simulink model "MotorDriveThermalTestbench"  (R2024b)
settings: Solver=daessc  StartTime=0.0  StopTime=2400  FixedStep=dt  RelTol=1e-3  AbsTol=1e-3
PreLoadFcn:
  | % Simulation parameters
  | MotorDriveThermalTestBenchParams;
model workspace (MAT data in the model file):
  V_frac_bridge = 0.0437
  V_fract_teeth = 0.9563
values from neighbouring files (symbols this model uses):
  CaseParams = struct()    [InverterThermalParams.m]
  HeatsinkParams = struct()    [InverterThermalParams.m]
undefined symbols (not defined in the file or in its folder): electricDrive, H_AH, H_AL, H_BH, H_BL, H_CH, H_CL, PipeParams, vehicleThermal
libraries: fl_lib x171, ee_lib x31, nesl_utility x28, nesl_utility_internal x12, sdl_lib x6, SimscapeFluids_lib x3, autolibshared x1
(part 2 of 4)

== system MotorDriveThermalTestbench/Motor Cooling/coolantJacket ==
  ControlTsump : fl_lib/Thermal Liquid/Elements/Reservoir (TL)  pressure_spec=foundation.enum.pressure_spec.atmospheric  reservoir_pressure=0.101325 MPa  reservoir_temperature=323.15 K  area=0.01 m^2
  Perfect Insulator : fl_lib/Thermal/Thermal Elements/Perfect Insulator  T_specify=off  T_priority=None  T=293.15 K  T_nominal_specify=off  T_nominal_value=1  T_nominal_unit=K
  Pipe : fl_lib/Thermal Liquid/Elements/Pipe (TL)  length=electricDrive.MotorThermal.ChannelLength mm  area=electricDrive.MotorThermal.ChannelSection mm^2  Dh=electricDrive.MotorThermal.ChannelHydraulicdia mm  length_add=500 mm  roughness=1.5e-5 m  Re_lam=2e+3  Re_tur=4e+3  shape_factor=64  Nu_lam=3.66  dynamic_compressibility=1  inertia=0  p0=1.1 atm  T0=323.15 K  mdot0=0.1 kg/s
  Pump : fl_lib/Thermal Liquid/Sources/Flow Rate Source (TL)  source_type=foundation.enum.constant_controlled.constant  flow_type=foundation.enum.mass_volumetric_flow.mass  mass_flow=pumpFlowRateM kg/s  volumetric_flow=0 m^3/s  power_spec=foundation.enum.power_spec.isentropic  area=pi*20^2 mm^2
      settings: InternalSimscapePortConfiguration="{\"Bottom\":[],\"Left\":[{\"id\":\"A\",\"label\":\"A\",\"type\":\"foundation.thermal_liquid.thermal_liquid\"}],\"Right\":[{\"id\":\"B\",\"label\":\"B\",\"type\":\"foundation.thermal_liquid.thermal_liquid\"}],\"Top\":[]}"
  Thermal Liquid Properties (TL) : SimscapeFluids_lib/Thermal Liquid/Utilities/Thermal Liquid Properties (TL)  fluid_list=fluids.thermal_liquid.utilities.enum.thermal_liquid_fluid_list.ethylene_glycol  concentration_param_EG=fluids.thermal_liquid.utilities.enum.thermal_liquid_concentration.volume_fraction  concentration_param_PG=fluids.thermal_liquid.utilities.enum.thermal_liquid_concentration.volume_fraction  c_mass_SW=3.5e-3  c_mass_EG=0.1  c_mass_PG=0.1  c_mass_GL=0.1  c_vol_EG=0.5  c_vol_PG=0.1  beta_const_EG=2.1791 GPa  beta_const_PG=2.1791 GPa  beta_const_GL=2.1791 GPa  p_min_EG=0.01 MPa  p_min_PG=0.01 MPa  p_min_GL=0.01 MPa  p_max_EG=50 MPa  p_max_PG=50 MPa  p_max_GL=50 MPa  p_atm=0.101325 MPa  properties_range_check=simscape.enum.assert.action.error
  JacketH : PMIOPort  Side=Left
  WindingH : PMIOPort  Port=2  Side=Left
  Ref : PMIOPort  Port=3  Side=Left
  connections:
  ControlTsump/LConn1 -- Thermal Liquid Properties (TL)/RConn1 -- Pump/LConn1
  Pipe/LConn2 -- JacketH/RConn1
  Pipe/RConn1 -- Pump/RConn1
  Pipe/LConn1 -- Ref/RConn1
  WindingH/RConn1 -- Perfect Insulator/LConn1

== system MotorDriveThermalTestbench/Motor Cooling/windingOilJet ==
  note: 1. Learn more about ThermalResistance submodel
  " oilflowRate " : fl_lib/Physical Signals/Sources/PS Constant  constant=electricDrive.MotorThermal.motorOilflow m^3/s
  Heat Exchanger (TL) : SimscapeFluids_lib/Heat Exchangers/Thermal Liquid/Heat Exchanger (TL)  hex_type=fluids.heat_exchangers.enum.FlowArrangement.ParallelCounter  shell_num=1  cross_type=fluids.heat_exchangers.enum.CrossFlowArrangementTL.MixedMixed  NTU_TLU=[.5, 1, 2, 3, 4, 5]  CR_TLU=[0, .25, .5, .75, 1]  eff_TLU=[.3, .3, .3, .3, .3; .6, .55, .5, .47, .43; .85, .76, .68, .61, .55; .94, .83, .72, .65, .58; .98, .86, .75, .66, .58; .99, .86, .75, .66, .58]  R_wall=1.6e-4 K/W  min_flow_area_1=0.01 m^2  Dh_press_1=0.1 m  liquid_volume_1=0.01 m^3  Re_lam_1=2000  Re_tur_1=4000  pressure_loss_spec_1=fluids.heat_exchangers.enum.PressureLossSpec.LossCoeff  pressure_loss_coeff_1=0.1  length_press_1=1 m  length_add_1=0.1 m  roughness_1=15e-6 m  Re_friction_TLU_1=[400, 1000, 1500, 3000, 4000, 6000, 10000, 20000, 40000, 60000, 100000, 100000000]  friction_factor_TLU_1=[.264, .112, .071, .0417, .0387, .0268, .025, .0232, .0226, .022, .0214, .0214]  shape_factor_1=64  Re_Euler_TLU_1=[50, 500, 1000, 2000]  Euler_TLU_1=[4.4505, .6864, .4791, .3755]  heat_transfer_spec_1=fluids.heat_exchangers.enum.HeatCoeffSpec.Constant  heat_transfer_area_1=0.4 m^2  heat_coeff_1=250 W/(K*m^2)  length_heat_1=1 m  Nu_lam_1=3.66  Re_Colburn_TLU_1=[100, 150, 1000]  Colburn_factor_TLU_1=[.019, .013, .002]  Re_Nu_TLU_1=[100, 150, 1000]  Pr_Nu_TLU_1=[1, 10]  Nu_TLU_1=[3.72, 4.21; 3.75, 4.44; 4.21, 7.15]  fouling_factor_1=1e-4 K*m^2/W  min_heat_coeff_1=5 W/(K*m^2)  heat_transfer_area_2=0.4 m^2  fouling_factor_2=1e-4 K*m^2/W  min_heat_coeff_2=5 W/(K*m^2)  dynamic_compressibility_1=simscape.enum.onoff.on  T0_1=298.15 K  p0_1=0.101325 MPa
      settings: InternalSimscapePortConfiguration="{\"Bottom\":[],\"Left\":[{\"id\":\"A1\",\"label\":\"A1\",\"type\":\"foundation.thermal_liquid.thermal_liquid\"},{\"id\":\"B1\",\"label\":\"B1\",\"type\":\"foundation.thermal_liquid.thermal_liquid\"}],\"Right\":[{\"id\":\"H2\",\"label\":\"H2\",\"type\":\"foundation.thermal.thermal\"},{\"id\":\"C2\",\"label\":\"C2\",\"type\":\"input\"},{\"id\":\"HC2\",\"label\":\"HC2\",\"type\":\"input\"}],\"Top\":[]}"
  HeatExHTC : fl_lib/Physical Signals/Sources/PS Constant  constant=300 W/(m^2*K)
  OilHeatCapacity : fl_lib/Physical Signals/Functions/PS Gain  gain=electricDrive.MotorThermal.oilDensity*electricDrive.MotorThermal.oilSpHeat J/(K*m^3)
  Perfect Insulator : fl_lib/Thermal/Thermal Elements/Perfect Insulator  T_specify=off  T_priority=None  T=293.15 K  T_nominal_specify=off  T_nominal_value=1  T_nominal_unit=K
  Pump : fl_lib/Thermal Liquid/Sources/Flow Rate Source (TL)  source_type=foundation.enum.constant_controlled.constant  flow_type=foundation.enum.mass_volumetric_flow.mass  mass_flow=pumpFlowRateM kg/s  volumetric_flow=0 m^3/s  power_spec=foundation.enum.power_spec.isentropic  area=pi*20^2 mm^2
      settings: InternalSimscapePortConfiguration="{\"Bottom\":[],\"Left\":[{\"id\":\"A\",\"label\":\"A\",\"type\":\"foundation.thermal_liquid.thermal_liquid\"}],\"Right\":[{\"id\":\"B\",\"label\":\"B\",\"type\":\"foundation.thermal_liquid.thermal_liquid\"}],\"Top\":[]}"
  Reservoir (TL) : fl_lib/Thermal Liquid/Elements/Reservoir (TL)  pressure_spec=foundation.enum.pressure_spec.atmospheric  reservoir_pressure=0.101325 MPa  reservoir_temperature=TankParams.Temp K  area=0.01 m^2
  Thermal Liquid Properties (TL) : SimscapeFluids_lib/Thermal Liquid/Utilities/Thermal Liquid Properties (TL)  fluid_list=fluids.thermal_liquid.utilities.enum.thermal_liquid_fluid_list.ethylene_glycol  concentration_param_EG=fluids.thermal_liquid.utilities.enum.thermal_liquid_concentration.volume_fraction  concentration_param_PG=fluids.thermal_liquid.utilities.enum.thermal_liquid_concentration.volume_fraction  c_mass_SW=3.5e-3  c_mass_EG=0.1  c_mass_PG=0.1  c_mass_GL=0.1  c_vol_EG=0.5  c_vol_PG=0.1  beta_const_EG=2.1791 GPa  beta_const_PG=2.1791 GPa  beta_const_GL=2.1791 GPa  p_min_EG=0.01 MPa  p_min_PG=0.01 MPa  p_min_GL=0.01 MPa  p_max_EG=50 MPa  p_max_PG=50 MPa  p_max_GL=50 MPa  p_atm=0.101325 MPa  properties_range_check=simscape.enum.assert.action.error
  "ThermalResistance " : Subsystem
      settings: PortSchema="{\"entries\":[{\"content\":{\"sides\":[{\"content\":{\"connectorIds\":[\"LConn1\",\"LConn2\"]},\"type\":\"ConnectorPlacement.EquallySpacedRectSide\",\"uuid\":\"baf5ff6f-2bbb-4e60-9dad-e00baf500c6c\"},{\"content\":{\"connectorIds\":[\"RConn1\"],\"side\":\"RIGHT\"},\"type\":\"ConnectorPlacement.EquallySpacedRectSide\",\"uuid\":\"04d231ab-fa8a-490b-9fb3-01902b632b73\"},{\"content\":{\"connectorIds\":[],\"side\":\"TOP\"},\"type\":\"ConnectorPlacement.EquallySpacedRectSide\",\"uuid\":\"736d11d8-afee-4ef0-b7ea-8bcbaef6669b\"},{\"content\":{\"connectorIds\":[\"RConn2\"],\"side\":\"BOTTOM\"},\"type\":\"ConnectorPlacement.EquallySpacedRectSide\",\"uuid\":\"7a09df8f-6346-484c-a8dd-3bdb74e2d22a\"}]},\"type\":\"ConnectorPlacement.EquallySpacedConnector\",\"uuid\":\"2b9b3d82-05b9-4b26-bdd0-141d56066ae3\"}],\"packageUris\":[\"http://schema.mathworks.com/mf0/Connector/R2020b\"],\"version\":\"1.0\"}"
      mask Display: image('$imagefile'); % Use "Edit Image" on toolstrip to change.
  Variable Thermal Resistance : fl_lib/Thermal/Thermal Elements/Variable Thermal Resistance  R_min=0 K/W  T_specify=off  T_priority=None  T=0 K  T_nominal_specify=off  T_nominal_value=1  T_nominal_unit=K  Q_specify=off  Q_priority=None  Q=0 W  Q_nominal_specify=off  Q_nominal_value=1  Q_nominal_unit=W
      settings: InternalSimscapePortConfiguration="{\"Bottom\":[],\"Left\":[{\"id\":\"A\",\"label\":\"A\",\"type\":\"foundation.thermal.thermal\"},{\"id\":\"R\",\"label\":\"R\",\"type\":\"input\"}],\"Right\":[{\"id\":\"B\",\"label\":\"B\",\"type\":\"foundation.thermal.thermal\"}],\"Top\":[]}"
  avgOilThickness : fl_lib/Physical Signals/Sources/PS Constant  constant=electricDrive.MotorThermal.Oft mm
  windingOD : fl_lib/Physical Signals/Sources/PS Constant  constant=electricDrive.MotorThermal.ODpcd*1e-3 m
  JacketH : PMIOPort  Side=Left
  WindingH : PMIOPort  Port=2  Side=Left
  Ref : PMIOPort  Port=3  Side=Left
  connections:
  Variable Thermal Resistance/RConn1 -- Heat Exchanger (TL)/RConn1
  Variable Thermal Resistance/LConn1 -- WindingH/RConn1
  " oilflowRate "/RConn1 -- OilHeatCapacity/LConn1 -- "ThermalResistance "/RConn2
  avgOilThickness/RConn1 -- "ThermalResistance "/LConn1
  windingOD/RConn1 -- "ThermalResistance "/LConn2
  Variable Thermal Resistance/LConn2 -- "ThermalResistance "/RConn1
  Ref/RConn1 -- Heat Exchanger (TL)/LConn2
  Reservoir (TL)/LConn1 -- Thermal Liquid Properties (TL)/RConn1 -- Pump/LConn1
  Pump/RConn1 -- Heat Exchanger (TL)/LConn1
  HeatExHTC/RConn1 -- Heat Exchanger (TL)/RConn3
  OilHeatCapacity/RConn1 -- Heat Exchanger (TL)/RConn2
  JacketH/RConn1 -- Perfect Insulator/LConn1

== system MotorDriveThermalTestbench/TemperatureLimits/Thermal fault Logic Inverter ==
  tc : Inport
  tm : Inport  Port=2
  CoilTempLimit : Constant  Value=IGBTlim
  Gain : Gain  OutDataTypeStr=double
  MagnetTempL imit : Constant  Value=DiodeLim
  MinMax : MinMax  Function=max  Inputs=2
  Relational Operator : RelationalOperator  OutDataTypeStr=boolean  RndMeth=Simplest  InputSameDT=off
  Relational Operator1 : RelationalOperator  OutDataTypeStr=boolean  RndMeth=Simplest  InputSameDT=off
  Unit Delay : UnitDelay  SampleTime=-1  HasFrameUpgradeWarning=on
  Unit Delay1 : UnitDelay  SampleTime=-1  HasFrameUpgradeWarning=on
  F : Outport
  wires:
  Relational Operator/1 -> MinMax/1
  MagnetTempL imit/1 -> Relational Operator1/2
  Relational Operator1/1 -> MinMax/2
  CoilTempLimit/1 -> Relational Operator/2
  Gain/1 -> F/1
  MinMax/1 -> Gain/1
  Unit Delay/1 -> Relational Operator/1
  tc/1 -> Unit Delay/1
  tm/1 -> Unit Delay1/1
  Unit Delay1/1 -> Relational Operator1/1

== system MotorDriveThermalTestbench/TemperatureLimits/Thermal fault Logic Motor ==
  tc : Inport
  tm : Inport  Port=2
  CoilTempLimit : Constant  Value=coilTLim
  Gain : Gain  OutDataTypeStr=double
  MagnetTempL imit : Constant  Value=MagTLim
  MinMax : MinMax  Function=max  Inputs=2
  Relational Operator : RelationalOperator  OutDataTypeStr=boolean  RndMeth=Simplest  InputSameDT=off
  Relational Operator1 : RelationalOperator  OutDataTypeStr=boolean  RndMeth=Simplest  InputSameDT=off
  Unit Delay : UnitDelay  SampleTime=-1  HasFrameUpgradeWarning=on
  Unit Delay1 : UnitDelay  SampleTime=-1  HasFrameUpgradeWarning=on
  F : Outport
  wires:
  Relational Operator/1 -> MinMax/1
  MagnetTempL imit/1 -> Relational Operator1/2
  Relational Operator1/1 -> MinMax/2
  CoilTempLimit/1 -> Relational Operator/2
  Gain/1 -> F/1
  MinMax/1 -> Gain/1
  Unit Delay/1 -> Relational Operator/1
  tc/1 -> Unit Delay/1
  tm/1 -> Unit Delay1/1
  Unit Delay1/1 -> Relational Operator1/1

== system MotorDriveThermalTestbench/Test Env N Controls/Motor speed N test environment ==
  VehSpd : Inport
  Motor Speed Reference : Subsystem
  Test Environment : Subsystem
  BrakeSig : Outport
  MtrSpdRef : Outport  Port=2
  wires:
  Test Environment/1(BrakeSig) -> BrakeSig/1
  VehSpd/1 -> Test Environment/1(tgtVspd), Motor Speed Reference/1(VSpd)
  Motor Speed Reference/1(MtrSpdRef) -> MtrSpdRef/1

== system MotorDriveThermalTestbench/Test Env N Controls/Speed Controller ==
  Spd : Inport  Unit=rpm
      settings: AttributesFormatString=%<Unit>
  SpdRef : Inport  Port=2  Unit=rpm
      settings: AttributesFormatString=%<Unit>
  Ki : Gain  Gain=electricDrive.PmsmControlParams.Kp_omega
  Kp : Gain  Gain=electricDrive.PmsmControlParams.Ki_omega
  Limits [-40,40] : Integrator  LimitOutput=on  UpperSaturationLimit=40  LowerSaturationLimit=-40
  Saturation : Saturate  UpperLimit=electricDrive.Tmax  LowerLimit=-electricDrive.Tmax
      settings: AttributesFormatString=|
      | %<UpperLimit>
      | %<LowerLimit>
  Sum : Sum  Inputs=-+|
  Sum1 : Sum  Inputs=++|
  Transfer Fcn : TransferFcn  Denominator=[0.1 1]
  TrqCmd : Outport  Unit=N*m  VectorParamsAs1DForOutWhenUnconnected=off
      settings: AttributesFormatString=%<Unit>
  wires:
  Saturation/1 -> TrqCmd/1
  Limits [-40,40]/1 -> Sum1/1
  Kp/1 -> Sum1/2
  Ki/1 -> Limits [-40,40]/1
  Sum/1 -> Kp/1, Ki/1
  Sum1/1 -> Saturation/1
  SpdRef/1 -> Sum/2
  Spd/1 -> Transfer Fcn/1
  Transfer Fcn/1 -> Sum/1

== system MotorDriveThermalTestbench/EM/Air_HTC_calculation/Rotor side  HTC ==
  PS Add : fl_lib/Physical Signals/Functions/PS Add
  PS Constant : fl_lib/Physical Signals/Sources/PS Constant  constant=8.1387 rad/s
  PS Gain1 : fl_lib/Physical Signals/Functions/PS Gain  gain=2.217 W*s/(m^2*K*rad)
  PS Gain2 : fl_lib/Physical Signals/Functions/PS Gain  gain=0.0265
  w : PMIOPort  Side=Left
  HTC : PMIOPort  Port=2  Side=Right
  connections:
  PS Constant/RConn1 -- PS Add/LConn2
  PS Gain2/RConn1 -- PS Add/LConn1
  PS Gain1/LConn1 -- PS Add/RConn1
  PS Gain1/RConn1 -- HTC/RConn1
  PS Gain2/LConn1 -- w/RConn1

== system MotorDriveThermalTestbench/EM/Air_HTC_calculation/Rotor_Taylor_Couette  HTC ==
  PS Add : fl_lib/Physical Signals/Functions/PS Add
  PS Constant : fl_lib/Physical Signals/Sources/PS Constant  constant=8.1387 rad/s
  PS Gain : fl_lib/Physical Signals/Functions/PS Gain  gain=2.667e-6 s/rad
  PS Gain1 : fl_lib/Physical Signals/Functions/PS Gain  gain=1 W/(m^2*K)
  PS Gain2 : fl_lib/Physical Signals/Functions/PS Gain  gain=0.0265
  PS-Simulink Converter : nesl_utility/PS-Simulink Converter  PhysicalDomain=network_engine_domain  SubClassName=ps_output  LeftPortType=input  RightPortType=output  PseudoPeriodic=off  Frequencies=[]  VectorFormat=inherit  Unit=inherit  AffineConversion=off
  Scope : Scope
  w : PMIOPort  Side=Left
  HTC_TC : PMIOPort  Port=2  Side=Right
  wires:
  PS-Simulink Converter/1 -> Scope/1
  connections:
  PS Add/RConn1 -- PS Gain/LConn1
  PS Constant/RConn1 -- PS Add/LConn2
  PS Gain2/RConn1 -- PS Add/LConn1
  HTC_TC/RConn1 -- PS-Simulink Converter/LConn1 -- PS Gain1/RConn1
  w/RConn1 -- PS Gain2/LConn1
  PS Gain/RConn1 -- PS Gain1/LConn1

== system MotorDriveThermalTestbench/EM/Loss Estimation/Copper Loss  ==
  PS Constant : fl_lib/Physical Signals/Sources/PS Constant  constant=0.0103 Ohm
  PS Gain : fl_lib/Physical Signals/Functions/PS Gain  gain=1
  PS Math Function : fl_lib/Physical Signals/Functions/PS Math Function  fcn_choice=foundation.enum.math_function.square  v=1
  PS Product : fl_lib/Physical Signals/Functions/PS Product
  Current : PMIOPort  Side=Left
  I2R : PMIOPort  Port=2  Side=Right
  connections:
  I2R/RConn1 -- PS Gain/RConn1
  PS Product/RConn1 -- PS Gain/LConn1
  PS Math Function/RConn1 -- PS Product/LConn1
  PS Constant/RConn1 -- PS Product/LConn2
  PS Math Function/LConn1 -- Current/RConn1

== system MotorDriveThermalTestbench/EM/Loss Estimation/Iron Loss ==
  PS Gain : fl_lib/Physical Signals/Functions/PS Gain  gain=electricDrive.MotorThermal.vFractBridge*0.4
  PS Gain1 : fl_lib/Physical Signals/Functions/PS Gain  gain=electricDrive.MotorThermal.vFractTooth*1.1
  PS Subtract : fl_lib/Physical Signals/Functions/PS Subtract
  MotH : PMIOPort  Side=Left
  I2R : PMIOPort  Port=2  Side=Left
  rt : PMIOPort  Port=3  Side=Right
  st : PMIOPort  Port=4  Side=Right
  connections:
  PS Gain1/RConn1 -- st/RConn1
  PS Gain/RConn1 -- rt/RConn1
  PS Gain1/LConn1 -- PS Gain/LConn1 -- PS Subtract/RConn1
  I2R/RConn1 -- PS Subtract/LConn2
  MotH/RConn1 -- PS Subtract/LConn1

== system MotorDriveThermalTestbench/EM/Loss Estimation/Subsystem ==
  Heat Flow Rate Sensor : fl_lib/Thermal/Thermal Sensors/Heat Flow Rate Sensor
  Temperature Source : fl_lib/Thermal/Thermal Sources/Temperature Source  temperature=298.15 K
  Hmot : PMIOPort  Side=Left
  MotH : PMIOPort  Port=2  Side=Right
  connections:
  Temperature Source/LConn1 -- Heat Flow Rate Sensor/RConn2
  Hmot/RConn1 -- Heat Flow Rate Sensor/LConn1
  MotH/RConn1 -- Heat Flow Rate Sensor/RConn1

== system MotorDriveThermalTestbench/EM/Subsystem1/Sensing wMotor ==
  PS-Simulink Converter : nesl_utility/PS-Simulink Converter  PhysicalDomain=network_engine_domain  SubClassName=ps_output  LeftPortType=input  RightPortType=output  PseudoPeriodic=off  Frequencies=[]  VectorFormat=1-D array  Unit=rpm  AffineConversion=off
  PS : PMIOPort  Side=Left
  SL : Outport  VectorParamsAs1DForOutWhenUnconnected=off
  wires:
  PS-Simulink Converter/1 -> SL/1
  connections:
  PS/RConn1 -- PS-Simulink Converter/LConn1

== system MotorDriveThermalTestbench/EM/Temperature/Bus ==
  Bus Creator : BusCreator  Inputs=2
  PS-Simulink Converter : nesl_utility/PS-Simulink Converter  PhysicalDomain=network_engine_domain  SubClassName=ps_output  LeftPortType=input  RightPortType=output  PseudoPeriodic=off  Frequencies=[]  VectorFormat=inherit  Unit=inherit  AffineConversion=off
  PS-Simulink Converter1 : nesl_utility/PS-Simulink Converter  PhysicalDomain=network_engine_domain  SubClassName=ps_output  LeftPortType=input  RightPortType=output  PseudoPeriodic=off  Frequencies=[]  VectorFormat=inherit  Unit=inherit  AffineConversion=off
  " " : PMIOPort  Side=Left
  "  " : PMIOPort  Port=2  Side=Left
  "   " : Outport
  wires:
  Bus Creator/1 -> "   "/1
  PS-Simulink Converter/1 -> Bus Creator/1  "Tmag"
  PS-Simulink Converter1/1 -> Bus Creator/2  "Tcoil"
  connections:
  " "/RConn1 -- PS-Simulink Converter/LConn1
  "  "/RConn1 -- PS-Simulink Converter1/LConn1

== system MotorDriveThermalTestbench/EM/Temperature/Rotor Thermal Block ==
  Conductive Heat Transfer : fl_lib/Thermal/Thermal Elements/Conductive Heat Transfer  thermal_type=foundation.enum.ConstantVariableTabulated.Constant  wall_geometry=foundation.enum.ConductionWallGeometry.Cylindrical  area=1e-4 m^2  thickness=0.1 m  d_in=0.005 m  d_out=rotor_od m  L=rotorStackLength m  th_cond_min=10 W/(K*m)  th_cond=IronThConductivity W/(K*m)  th_cond_TLU=[413, 401, 392, 383, 371, 357, 342] W/(K*m)  temp_TLU=[200, 273, 400, 600, 800, 1000, 1200] K  T_specify=off  T_priority=None  T=0 K  T_nominal_specify=off  T_nominal_value=1  T_nominal_unit=K  Q_specify=off  Q_priority=None  Q=0 W  Q_nominal_specify=off  Q_nominal_value=1  Q_nominal_unit=W
  Convective Heat Transfer : fl_lib/Thermal/Thermal Elements/Convective Heat Transfer  thermal_type=foundation.enum.constant_variable.variable  area=RotorAreaCyl m^2  heat_tr_coeff=10 W/(K*m^2)  min_heat_tr_coeff=1e-3 W/(K*m^2)  T_specify=off  T_priority=None  T=0 K  T_nominal_specify=off  T_nominal_value=1  T_nominal_unit=K  Q_specify=off  Q_priority=None  Q=0 W  Q_nominal_specify=off  Q_nominal_value=1  Q_nominal_unit=W
      settings: InternalSimscapePortConfiguration="{\"Bottom\":[],\"Left\":[{\"id\":\"A\",\"label\":\"A\",\"type\":\"foundation.thermal.thermal\"},{\"id\":\"var_heat_tr_coeff\",\"label\":\"K\",\"type\":\"input\"}],\"Right\":[{\"id\":\"B\",\"label\":\"B\",\"type\":\"foundation.thermal.thermal\"}],\"Top\":[]}"
  Convective Heat Transfer1 : fl_lib/Thermal/Thermal Elements/Convective Heat Transfer  thermal_type=foundation.enum.constant_variable.variable  area=RotorAreaER m^2  heat_tr_coeff=20 W/(K*m^2)  min_heat_tr_coeff=1e-3 W/(K*m^2)  T_specify=off  T_priority=None  T=0 K  T_nominal_specify=off  T_nominal_value=1  T_nominal_unit=K  Q_specify=off  Q_priority=None  Q=0 W  Q_nominal_specify=off  Q_nominal_value=1  Q_nominal_unit=W
      settings: InternalSimscapePortConfiguration="{\"Bottom\":[],\"Left\":[{\"id\":\"A\",\"label\":\"A\",\"type\":\"foundation.thermal.thermal\"},{\"id\":\"var_heat_tr_coeff\",\"label\":\"K\",\"type\":\"input\"}],\"Right\":[{\"id\":\"B\",\"label\":\"B\",\"type\":\"foundation.thermal.thermal\"}],\"Top\":[]}"
  Heat Flow Source : fl_lib/Thermal/Thermal Sources/Controlled Heat Flow Rate Source
  "Magnet_Temperature " : fl_lib/Thermal/Thermal Elements/Thermal Mass  mass_type=foundation.enum.constant_variable.constant  mass=Bridgemass kg  sp_heat=IronSpHeat J/(K*kg)  mass_min=1e-6 kg  num_ports=foundation.enum.numPorts2.one  m_specify=off  m_priority=High  m=1 kg  m_nominal_specify=off  m_nominal_value=1  m_nominal_unit=kg  T_specify=on  T_priority=High  T=InitTemp K  T_nominal_specify=off  T_nominal_value=1  T_nominal_unit=K  Q_specify=off  Q_priority=None  Q=0 W  Q_nominal_specify=off  Q_nominal_value=1  Q_nominal_unit=W
  MotorHousingTemperature : fl_lib/Thermal/Thermal Sources/Temperature Source  temperature=90 degC
  Rotor Back Iron : fl_lib/Thermal/Thermal Elements/Thermal Mass  mass_type=foundation.enum.constant_variable.constant  mass=RotorBackIronMass kg  sp_heat=IronSpHeat J/(K*kg)  mass_min=1e-6 kg  num_ports=foundation.enum.numPorts2.one  m_specify=off  m_priority=High  m=1 kg  m_nominal_specify=off  m_nominal_value=1  m_nominal_unit=kg  T_specify=on  T_priority=High  T=InitTemp K  T_nominal_specify=off  T_nominal_value=1  T_nominal_unit=K  Q_specify=off  Q_priority=None  Q=0 W  Q_nominal_specify=off  Q_nominal_value=1  Q_nominal_unit=W
  Sensor : Subsystem
  Thermal Reference : fl_lib/Thermal/Thermal Elements/Thermal Reference
  H_rot : PMIOPort  Side=Right
  HTC_AG : PMIOPort  Port=2  Side=Right
  HTC_ER : PMIOPort  Port=3  Side=Right
  Magnet Temp : PMIOPort  Port=4  Side=Left
  connections:
  Magnet Temp/RConn1 -- Sensor/RConn1
  H_rot/RConn1 -- Heat Flow Source/RConn1
  HTC_ER/RConn1 -- Convective Heat Transfer1/LConn2
  HTC_AG/RConn1 -- Convective Heat Transfer/LConn2
  Convective Heat Transfer/LConn1 -- Sensor/LConn1 -- Conductive Heat Transfer/LConn1 -- "Magnet_Temperature "/LConn1 -- Heat Flow Source/LConn1
  MotorHousingTemperature/LConn1 -- Convective Heat Transfer1/RConn1 -- Convective Heat Transfer/RConn1
  Rotor Back Iron/LConn1 -- Convective Heat Transfer1/LConn1 -- Conductive Heat Transfer/RConn1
  Thermal Reference/LConn1 -- Heat Flow Source/RConn2

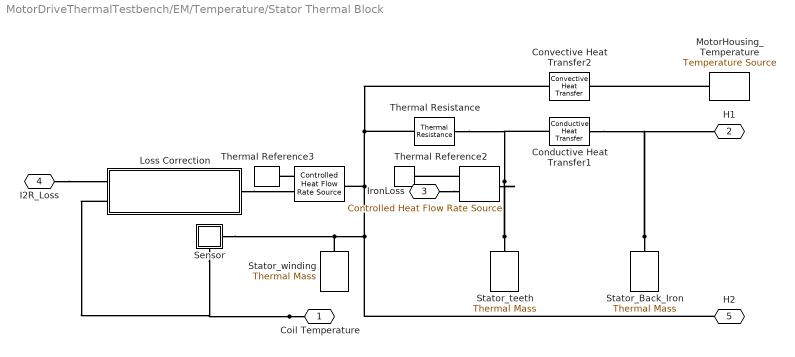
== system MotorDriveThermalTestbench/EM/Temperature/Stator Thermal Block ==
  " " : fl_lib/Thermal/Thermal Sources/Controlled Heat Flow Rate Source
  "  " : fl_lib/Thermal/Thermal Sources/Controlled Heat Flow Rate Source
  Conductive Heat Transfer1 : fl_lib/Thermal/Thermal Elements/Conductive Heat Transfer  thermal_type=foundation.enum.ConstantVariableTabulated.Constant  wall_geometry=foundation.enum.ConductionWallGeometry.Cylindrical  area=1e-4 m^2  thickness=0.1 m  d_in=StatorRootDia m  d_out=stator_od m  L=rotorStackLength m  th_cond_min=10 W/(K*m)  th_cond=50 W/(K*m)  th_cond_TLU=[413, 401, 392, 383, 371, 357, 342] W/(K*m)  temp_TLU=[200, 273, 400, 600, 800, 1000, 1200] K  T_specify=off  T_priority=None  T=0 K  T_nominal_specify=off  T_nominal_value=1  T_nominal_unit=K  Q_specify=off  Q_priority=None  Q=0 W  Q_nominal_specify=off  Q_nominal_value=1  Q_nominal_unit=W
  Convective Heat Transfer2 : fl_lib/Thermal/Thermal Elements/Convective Heat Transfer  thermal_type=foundation.enum.constant_variable.constant  area=StatorWindingOhArea m^2  heat_tr_coeff=1 W/(K*m^2)  min_heat_tr_coeff=1e-3 W/(K*m^2)  T_specify=off  T_priority=None  T=0 K  T_nominal_specify=off  T_nominal_value=1  T_nominal_unit=K  Q_specify=off  Q_priority=None  Q=0 W  Q_nominal_specify=off  Q_nominal_value=1  Q_nominal_unit=W
  Loss Correction : Subsystem
  MotorHousing_Temperature : fl_lib/Thermal/Thermal Sources/Temperature Source  temperature=90 degC
  Sensor : Subsystem
      settings: PortSchema="{\"entries\":[{\"content\":{\"sides\":[{\"content\":{\"connectorIds\":[\"LConn1\"]},\"type\":\"ConnectorPlacement.EquallySpacedRectSide\",\"uuid\":\"2a9c4c46-5e98-4ad3-ac1b-1643fab919e9\"},{\"content\":{\"connectorIds\":[],\"side\":\"RIGHT\"},\"type\":\"ConnectorPlacement.EquallySpacedRectSide\",\"uuid\":\"818e06c0-624d-478e-bbcc-fcb04ee6018d\"},{\"content\":{\"connectorIds\":[],\"side\":\"TOP\"},\"type\":\"ConnectorPlacement.EquallySpacedRectSide\",\"uuid\":\"5528f141-53ee-42de-bb84-2bf943b57dce\"},{\"content\":{\"connectorIds\":[\"RConn1\"],\"side\":\"BOTTOM\"},\"type\":\"ConnectorPlacement.EquallySpacedRectSide\",\"uuid\":\"84eb734e-86a3-4614-b5bf-5af47052b8ad\"}]},\"type\":\"ConnectorPlacement.EquallySpacedConnector\",\"uuid\":\"b22b55cd-2470-4ac9-8f94-59072ebe807a\"}],\"packageUris\":[\"http://schema.mathworks.com/mf0/Connector/R2020b\"],\"version\":\"1.0\"}"
  Stator_Back_Iron : fl_lib/Thermal/Thermal Elements/Thermal Mass  mass_type=foundation.enum.constant_variable.constant  mass=StatorBackIronMass kg  sp_heat=IronSpHeat J/(K*kg)  mass_min=1e-6 kg  num_ports=foundation.enum.numPorts2.one  m_specify=off  m_priority=High  m=1 kg  m_nominal_specify=off  m_nominal_value=1  m_nominal_unit=kg  T_specify=on  T_priority=High  T=InitTemp K  T_nominal_specify=off  T_nominal_value=1  T_nominal_unit=K  Q_specify=off  Q_priority=None  Q=0 W  Q_nominal_specify=off  Q_nominal_value=1  Q_nominal_unit=W
  Stator_teeth : fl_lib/Thermal/Thermal Elements/Thermal Mass  mass_type=foundation.enum.constant_variable.constant  mass=GrossToothMass kg  sp_heat=IronSpHeat J/(K*kg)  mass_min=1e-6 kg  num_ports=foundation.enum.numPorts2.one  m_specify=off  m_priority=High  m=1 kg  m_nominal_specify=off  m_nominal_value=1  m_nominal_unit=kg  T_specify=on  T_priority=High  T=InitTemp K  T_nominal_specify=off  T_nominal_value=1  T_nominal_unit=K  Q_specify=off  Q_priority=None  Q=0 W  Q_nominal_specify=off  Q_nominal_value=1  Q_nominal_unit=W
  Stator_winding : fl_lib/Thermal/Thermal Elements/Thermal Mass  mass_type=foundation.enum.constant_variable.constant  mass=WindingMass kg  sp_heat=CopperSpHeat J/(K*kg)  mass_min=1e-6 kg  num_ports=foundation.enum.numPorts2.one  m_specify=off  m_priority=High  m=1 kg  m_nominal_specify=off  m_nominal_value=1  m_nominal_unit=kg  T_specify=on  T_priority=High  T=InitTemp K  T_nominal_specify=off  T_nominal_value=1  T_nominal_unit=K  Q_specify=off  Q_priority=None  Q=0 W  Q_nominal_specify=off  Q_nominal_value=1  Q_nominal_unit=W
  Thermal Reference2 : fl_lib/Thermal/Thermal Elements/Thermal Reference
  Thermal Reference3 : fl_lib/Thermal/Thermal Elements/Thermal Reference
  Thermal Resistance : fl_lib/Thermal/Thermal Elements/Thermal Resistance  resistance=0.1 K/W  T_specify=off  T_priority=None  T=0 K  T_nominal_specify=off  T_nominal_value=1  T_nominal_unit=K  Q_specify=off  Q_priority=None  Q=0 W  Q_nominal_specify=off  Q_nominal_value=1  Q_nominal_unit=W
  Coil Temperature : PMIOPort  Side=Left
  H1 : PMIOPort  Port=2  Side=Left
  IronLoss : PMIOPort  Port=3  Side=Right
  I2R_Loss : PMIOPort  Port=4  Side=Right
  H2 : PMIOPort  Port=5  Side=Left
  connections:
  I2R_Loss/RConn1 -- Loss Correction/LConn1
  Coil Temperature/RConn1 -- Loss Correction/LConn2 -- Sensor/LConn1
  Loss Correction/RConn1 -- "  "/RConn1
  IronLoss/RConn1 -- " "/RConn1
  " "/RConn2 -- Thermal Reference2/LConn1
  "  "/RConn2 -- Thermal Reference3/LConn1
  MotorHousing_Temperature/LConn1 -- Convective Heat Transfer2/RConn1
  Sensor/RConn1 -- "  "/LConn1 -- Thermal Resistance/RConn1 -- Convective Heat Transfer2/LConn1 -- H2/RConn1 -- Stator_winding/LConn1
  Stator_teeth/LConn1 -- Thermal Resistance/LConn1 -- Conductive Heat Transfer1/LConn1 -- " "/LConn1
  Stator_Back_Iron/LConn1 -- H1/RConn1 -- Conductive Heat Transfer1/RConn1

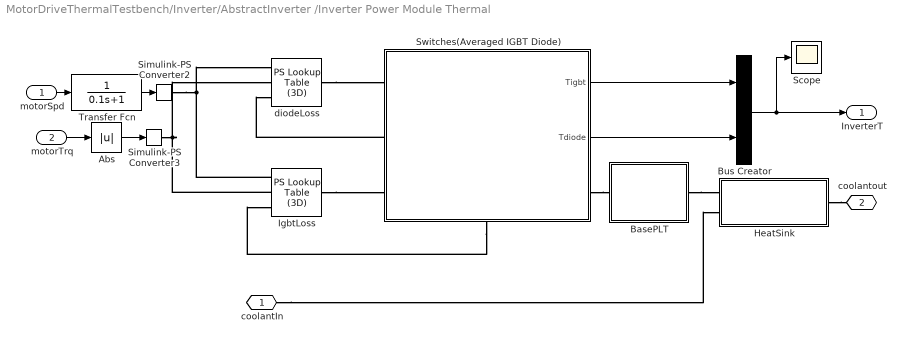
== system MotorDriveThermalTestbench/Inverter/AbstractInverter /Inverter Power Module Thermal ==
  motorSpd : Inport
  motorTrq : Inport  Port=2
  Abs : Abs  SaturateOnIntegerOverflow=off
  BasePLT : Subsystem
  Bus Creator : BusCreator  Inputs=2
  HeatSink : Subsystem
  IgbtLoss : fl_lib/Physical Signals/Lookup Tables/PS Lookup Table (3D)  x1=electricDrive.motor_loss_map.spMat rpm  x2=electricDrive.motor_loss_map.tqMat N*m  x3=[25,125, 175]+273.15 K  f=electricDrive.inverter_loss_map.lossMatIgbt  interp_method=simscape.enum.interpolation.linear  extrap_method=simscape.enum.extrapolation.linear
      settings: InternalSimscapePortConfiguration="{\"Bottom\":[],\"Left\":[{\"id\":\"I1\",\"label\":\"x1\",\"type\":\"input\"},{\"id\":\"I2\",\"label\":\"x2\",\"type\":\"input\"},{\"id\":\"I3\",\"label\":\"x3\",\"type\":\"input\"}],\"Right\":[{\"id\":\"O\",\"label\":\"f\",\"type\":\"output\"}],\"Top\":[]}"
  Scope : Scope
  Simulink-PS Converter2 : nesl_utility/Simulink-PS Converter  PhysicalDomain=network_engine_domain  SubClassName=ps_input  LeftPortType=input  RightPortType=output  PseudoPeriodic=off  Frequencies=[]  NoiseDistribution=none  NoiseParameters=[]  Unit=rpm  AffineConversion=off  FilteringAndDerivatives=provide  SimscapeFilterOrder=1  InputFilterTimeConstant=0.001  UdotUserProvided=0
  Simulink-PS Converter3 : nesl_utility/Simulink-PS Converter  PhysicalDomain=network_engine_domain  SubClassName=ps_input  LeftPortType=input  RightPortType=output  PseudoPeriodic=off  Frequencies=[]  NoiseDistribution=none  NoiseParameters=[]  Unit=N*m  AffineConversion=off  FilteringAndDerivatives=provide  SimscapeFilterOrder=1  InputFilterTimeConstant=0.001  UdotUserProvided=0
  Switches(Averaged IGBT Diode) : Subsystem
      settings: PortSchema="{\"entries\":[{\"content\":{\"sides\":[{\"content\":{\"connectorIds\":[\"Out1\",\"Out2\",\"LConn1\"]},\"type\":\"ConnectorPlacement.EquallySpacedRectSide\",\"uuid\":\"c466717f-a559-4c42-b6dd-2de508982627\"},{\"content\":{\"connectorIds\":[\"RConn1\",\"RConn2\",\"RConn3\"],\"side\":\"RIGHT\"},\"type\":\"ConnectorPlacement.EquallySpacedRectSide\",\"uuid\":\"5a44429a-0c01-47a4-96c4-89a03d92af2a\"},{\"content\":{\"connectorIds\":[],\"side\":\"TOP\"},\"type\":\"ConnectorPlacement.EquallySpacedRectSide\",\"uuid\":\"592797f6-2176-45a1-8a5a-ffba72eaaa30\"},{\"content\":{\"connectorIds\":[\"RConn4\"],\"side\":\"BOTTOM\"},\"type\":\"ConnectorPlacement.EquallySpacedRectSide\",\"uuid\":\"45f39216-5c54-48d4-857b-159bfbffda40\"}]},\"type\":\"ConnectorPlacement.EquallySpacedConnector\",\"uuid\":\"8211d252-7bec-4c59-be39-60a0fcf206ce\"}],\"packageUris\":[\"http://schema.mathworks.com/mf0/Connector/R2020b\"],\"version\":\"1.0\"}"
      mask Display: image('$imagefile'); % Use "Edit Image" on toolstrip to change.
  Transfer Fcn : TransferFcn  Denominator=[0.1 1]
  diodeLoss : fl_lib/Physical Signals/Lookup Tables/PS Lookup Table (3D)  x1=electricDrive.motor_loss_map.spMat rpm  x2=electricDrive.motor_loss_map.tqMat N*m  x3=[25,125, 175]+273.15 K  f=electricDrive.inverter_loss_map.lossMatDiode  interp_method=simscape.enum.interpolation.linear  extrap_method=simscape.enum.extrapolation.linear
      settings: InternalSimscapePortConfiguration="{\"Bottom\":[],\"Left\":[{\"id\":\"I1\",\"label\":\"x1\",\"type\":\"input\"},{\"id\":\"I2\",\"label\":\"x2\",\"type\":\"input\"},{\"id\":\"I3\",\"label\":\"x3\",\"type\":\"input\"}],\"Right\":[{\"id\":\"O\",\"label\":\"f\",\"type\":\"output\"}],\"Top\":[]}"
  coolantIn : PMIOPort  Side=Left
  coolantout : PMIOPort  Port=2  Side=Right
  InverterT : Outport
  wires:
  Switches(Averaged IGBT Diode)/1(Tigbt) -> Bus Creator/1
  Switches(Averaged IGBT Diode)/2(Tdiode) -> Bus Creator/2
  Bus Creator/1 -> Scope/1, InverterT/1
  motorTrq/1 -> Abs/1
  motorSpd/1 -> Transfer Fcn/1
  Abs/1 -> Simulink-PS Converter3/1
  Transfer Fcn/1 -> Simulink-PS Converter2/1
  connections:
  IgbtLoss/RConn1 -- Switches(Averaged IGBT Diode)/RConn3
  diodeLoss/RConn1 -- Switches(Averaged IGBT Diode)/RConn1
  IgbtLoss/LConn1 -- diodeLoss/LConn1 -- Simulink-PS Converter2/RConn1
  IgbtLoss/LConn2 -- Simulink-PS Converter3/RConn1 -- diodeLoss/LConn2
  Switches(Averaged IGBT Diode)/RConn2 -- diodeLoss/LConn3
  Switches(Averaged IGBT Diode)/RConn4 -- IgbtLoss/LConn3
  BasePLT/RConn1 -- HeatSink/LConn1
  Switches(Averaged IGBT Diode)/LConn1 -- BasePLT/LConn1
  coolantIn/RConn1 -- HeatSink/LConn2
  HeatSink/RConn1 -- coolantout/RConn1

== system MotorDriveThermalTestbench/Inverter/DetailedInverter/BaseplateAndHeatsink ==
  BasePLT : Subsystem
      settings: PortSchema="{\"entries\":[{\"content\":{\"sides\":[{\"content\":{\"connectorIds\":[\"LConn1\"]},\"type\":\"ConnectorPlacement.EquallySpacedRectSide\",\"uuid\":\"06bea180-76e4-485f-8c92-98df5c260dca\"},{\"content\":{\"connectorIds\":[\"RConn1\",\"RConn2\",\"RConn3\"],\"side\":\"RIGHT\"},\"type\":\"ConnectorPlacement.EquallySpacedRectSide\",\"uuid\":\"a99e02fc-6b0a-45f4-a178-f59447542951\"},{\"content\":{\"connectorIds\":[\"Out1\"],\"side\":\"TOP\"},\"type\":\"ConnectorPlacement.EquallySpacedRectSide\",\"uuid\":\"22e7057d-114f-4fd7-9900-45601d3a5816\"},{\"content\":{\"connectorIds\":[],\"side\":\"BOTTOM\"},\"type\":\"ConnectorPlacement.EquallySpacedRectSide\",\"uuid\":\"03812fa4-5872-4b87-bc29-7e84d74c14de\"}]},\"type\":\"ConnectorPlacement.EquallySpacedConnector\",\"uuid\":\"fb67c2f1-41fe-4b38-a14a-a438a4403cb8\"}],\"packageUris\":[\"http://schema.mathworks.com/mf0/Connector/R2020b\"],\"version\":\"1.0\"}"
  HeatSink : Subsystem
      settings: PortSchema="{\"entries\":[{\"content\":{\"sides\":[{\"content\":{\"connectorIds\":[\"LConn1\"]},\"type\":\"ConnectorPlacement.EquallySpacedRectSide\",\"uuid\":\"c35c2cca-88c8-49f3-81d6-30e8c5a69bc3\"},{\"content\":{\"connectorIds\":[\"RConn1\"],\"side\":\"RIGHT\"},\"type\":\"ConnectorPlacement.EquallySpacedRectSide\",\"uuid\":\"81cb188b-caaf-40f1-ac11-54d241445da6\"},{\"content\":{\"connectorIds\":[\"LConn2\",\"LConn3\",\"LConn4\"],\"side\":\"TOP\"},\"type\":\"ConnectorPlacement.EquallySpacedRectSide\",\"uuid\":\"6380ff7a-628b-4735-8746-e0e816d8feed\"}]},\"type\":\"ConnectorPlacement.EquallySpacedConnector\",\"uuid\":\"be9b966f-9b78-4c1a-8fd2-410f7c811f74\"}],\"packageUris\":[\"http://schema.mathworks.com/mf0/Connector/R2020b\"],\"version\":\"1.0\"}"
      mask Display: image('$imagefile'); % Use "Edit Image" on toolstrip to change.
  Inlet : PMIOPort  Side=Left
  Hc : PMIOPort  Port=2  Side=Left
  Outlet : PMIOPort  Port=3  Side=Right
  Tc : Outport
  wires:
  BasePLT/1(Tmeas) -> Tc/1
  connections:
  BasePLT/RConn2 -- HeatSink/LConn3
  BasePLT/RConn1 -- HeatSink/LConn4
  Outlet/RConn1 -- HeatSink/RConn1
  BasePLT/RConn3 -- HeatSink/LConn2
  Inlet/RConn1 -- HeatSink/LConn1
  Hc/RConn1 -- BasePLT/LConn1

== system MotorDriveThermalTestbench/Inverter/DetailedInverter/PowerLoss ==
  mspd : Inport
  tq : Inport  Port=2
  Tdiode : Inport  Port=3
  Tigbt : Inport  Port=4
  DiodeLoss : Subsystem
  IGBTloss : Subsystem
  Higbt : Outport
  Hdiode : Outport  Port=2
  wires:
  IGBTloss/1(loss) -> Higbt/1
  tq/1 -> IGBTloss/2(mtq), DiodeLoss/1(mtq)
  DiodeLoss/1(Hloss) -> Hdiode/1
  Tigbt/1 -> IGBTloss/3(temp)
  mspd/1 -> IGBTloss/1(mspd), DiodeLoss/2(mspd)
  Tdiode/1 -> DiodeLoss/3(temp)

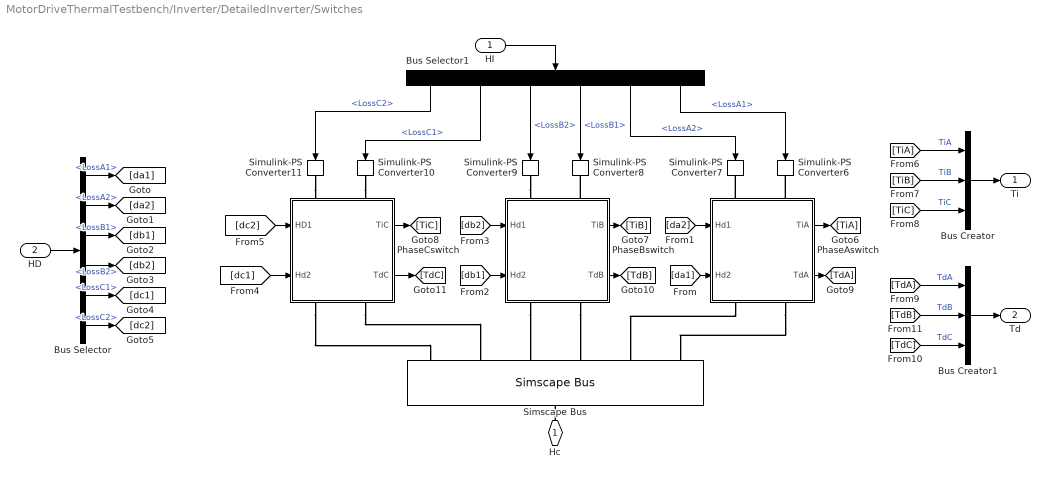
== system MotorDriveThermalTestbench/Inverter/DetailedInverter/Switches ==
  HI : Inport
  HD : Inport  Port=2
  Bus Creator : BusCreator  Inputs=3
  Bus Creator1 : BusCreator  Inputs=3
  Bus Selector : BusSelector  OutputSignals=LossA1,LossA2,LossB1,LossB2,LossC1,LossC2
  Bus Selector1 : BusSelector  OutputSignals=LossC2,LossC1,LossB2,LossB1,LossA2,LossA1
  PhaseAswitch : Subsystem
      settings: PortSchema="{\"entries\":[{\"content\":{\"sides\":[{\"content\":{\"connectorIds\":[\"LConn1\",\"LConn2\"]},\"type\":\"ConnectorPlacement.EquallySpacedRectSide\",\"uuid\":\"5f7affab-94ba-4b7f-a148-0a32bfd918ba\"},{\"content\":{\"connectorIds\":[\"RConn1\",\"RConn2\"],\"side\":\"RIGHT\"},\"type\":\"ConnectorPlacement.EquallySpacedRectSide\",\"uuid\":\"63d9d7a2-362e-4409-8a34-3b6dc92bbacd\"},{\"content\":{\"connectorIds\":[\"In1\",\"In2\"],\"side\":\"TOP\"},\"type\":\"ConnectorPlacement.EquallySpacedRectSide\",\"uuid\":\"c6a1408d-ff32-45b0-a0a7-c7b458ab5913\"},{\"content\":{\"connectorIds\":[\"Out1\",\"Out2\"],\"side\":\"BOTTOM\"},\"type\":\"ConnectorPlacement.EquallySpacedRectSide\",\"uuid\":\"3724aedb-33ec-497c-bd76-22af29b532da\"}]},\"type\":\"ConnectorPlacement.EquallySpacedConnector\",\"uuid\":\"16c665ab-3f5c-4f9c-81fe-dd0c56427ac7\"}],\"packageUris\":[\"http://schema.mathworks.com/mf0/Connector/R2020b\"],\"version\":\"1.0\"}"
      mask Display: image('$imagefile'); % Use "Edit Image" on toolstrip to change.
  PhaseBswitch : Subsystem
      settings: PortSchema="{\"entries\":[{\"content\":{\"sides\":[{\"content\":{\"connectorIds\":[\"LConn1\",\"LConn2\"]},\"type\":\"ConnectorPlacement.EquallySpacedRectSide\",\"uuid\":\"5f7affab-94ba-4b7f-a148-0a32bfd918ba\"},{\"content\":{\"connectorIds\":[\"RConn1\",\"RConn2\"],\"side\":\"RIGHT\"},\"type\":\"ConnectorPlacement.EquallySpacedRectSide\",\"uuid\":\"63d9d7a2-362e-4409-8a34-3b6dc92bbacd\"},{\"content\":{\"connectorIds\":[\"In1\",\"In2\"],\"side\":\"TOP\"},\"type\":\"ConnectorPlacement.EquallySpacedRectSide\",\"uuid\":\"c6a1408d-ff32-45b0-a0a7-c7b458ab5913\"},{\"content\":{\"connectorIds\":[\"Out1\",\"Out2\"],\"side\":\"BOTTOM\"},\"type\":\"ConnectorPlacement.EquallySpacedRectSide\",\"uuid\":\"fa987dc5-6284-4113-a899-b0034d7fba99\"}]},\"type\":\"ConnectorPlacement.EquallySpacedConnector\",\"uuid\":\"16c665ab-3f5c-4f9c-81fe-dd0c56427ac7\"}],\"packageUris\":[\"http://schema.mathworks.com/mf0/Connector/R2020b\"],\"version\":\"1.0\"}"
      mask Display: image('$imagefile'); % Use "Edit Image" on toolstrip to change.
  PhaseCswitch : Subsystem
      settings: PortSchema="{\"entries\":[{\"content\":{\"sides\":[{\"content\":{\"connectorIds\":[\"LConn1\",\"LConn2\"]},\"type\":\"ConnectorPlacement.EquallySpacedRectSide\",\"uuid\":\"5f7affab-94ba-4b7f-a148-0a32bfd918ba\"},{\"content\":{\"connectorIds\":[\"RConn1\",\"RConn2\"],\"side\":\"RIGHT\"},\"type\":\"ConnectorPlacement.EquallySpacedRectSide\",\"uuid\":\"63d9d7a2-362e-4409-8a34-3b6dc92bbacd\"},{\"content\":{\"connectorIds\":[\"In1\",\"In2\"],\"side\":\"TOP\"},\"type\":\"ConnectorPlacement.EquallySpacedRectSide\",\"uuid\":\"c6a1408d-ff32-45b0-a0a7-c7b458ab5913\"},{\"content\":{\"connectorIds\":[\"Out1\",\"Out2\"],\"side\":\"BOTTOM\"},\"type\":\"ConnectorPlacement.EquallySpacedRectSide\",\"uuid\":\"d8fa1913-6c6d-48c0-812a-ccf51817ee73\"}]},\"type\":\"ConnectorPlacement.EquallySpacedConnector\",\"uuid\":\"16c665ab-3f5c-4f9c-81fe-dd0c56427ac7\"}],\"packageUris\":[\"http://schema.mathworks.com/mf0/Connector/R2020b\"],\"version\":\"1.0\"}"
      mask Display: image('$imagefile'); % Use "Edit Image" on toolstrip to change.
  Simscape Bus : SimscapeBus  HierarchyStrings=H_CL;H_CH;H_BL;H_BH;H_AL;H_AH
  Simulink-PS Converter{6..11} (6 alike) : nesl_utility/Simulink-PS Converter  PhysicalDomain=network_engine_domain  SubClassName=ps_input  LeftPortType=input  RightPortType=output  PseudoPeriodic=off  Frequencies=[]  NoiseDistribution=none  NoiseParameters=[]  Unit=J/s  AffineConversion=off  FilteringAndDerivatives=provide  SimscapeFilterOrder=1  InputFilterTimeConstant=0.001  UdotUserProvided=0
  Hc : PMIOPort  Tag=PMCPort  Side=Right
  Ti : Outport
  Td : Outport  Port=2
  wires:
  HD/1 -> Bus Selector/1
  Bus Selector/1 -> [da1]  "<LossA1>"
  Bus Selector/2 -> [da2]  "<LossA2>"
  Bus Selector/3 -> [db1]  "<LossB1>"
  Bus Selector/4 -> [db2]  "<LossB2>"
  Bus Selector/5 -> [dc1]  "<LossC1>"
  Bus Selector/6 -> [dc2]  "<LossC2>"
  HI/1 -> Bus Selector1/1
  Bus Selector1/6 -> Simulink-PS Converter6/1  "<LossA1>"
  Bus Selector1/1 -> Simulink-PS Converter11/1  "<LossC2>"
  Bus Selector1/2 -> Simulink-PS Converter10/1  "<LossC1>"
  Bus Selector1/3 -> Simulink-PS Converter9/1  "<LossB2>"
  Bus Selector1/4 -> Simulink-PS Converter8/1  "<LossB1>"
  Bus Selector1/5 -> Simulink-PS Converter7/1  "<LossA2>"
  Bus Creator/1 -> Ti/1
  Bus Creator1/1 -> Td/1
  [da1] -> PhaseAswitch/1(Hd2)
  [da2] -> PhaseAswitch/2(Hd1)
  [db1] -> PhaseBswitch/1(Hd2)
  [db2] -> PhaseBswitch/2(Hd1)
  [dc1] -> PhaseCswitch/1(Hd2)
  [dc2] -> PhaseCswitch/2(HD1)
  PhaseBswitch/2(TiB) -> [TiB]
  PhaseCswitch/2(TiC) -> [TiC]
  PhaseAswitch/2(TiA) -> [TiA]
  PhaseAswitch/1(TdA) -> [TdA]
  PhaseBswitch/1(TdB) -> [TdB]
  PhaseCswitch/1(" TdC") -> [TdC]
  [TiA] -> Bus Creator/1  "TiA"
  [TiB] -> Bus Creator/2  "TiB"
  [TiC] -> Bus Creator/3  "TiC"
  [TdA] -> Bus Creator1/1  "TdA"
  [TdB] -> Bus Creator1/2  "TdB"
  [TdC] -> Bus Creator1/3  "TdC"
  connections:
  Hc/RConn1 -- Simscape Bus/RConn1
  PhaseAswitch/RConn2 -- Simulink-PS Converter6/RConn1
  PhaseAswitch/RConn1 -- Simulink-PS Converter7/RConn1
  PhaseBswitch/RConn2 -- Simulink-PS Converter8/RConn1
  Simulink-PS Converter9/RConn1 -- PhaseBswitch/RConn1
  Simulink-PS Converter10/RConn1 -- PhaseCswitch/RConn2
  Simulink-PS Converter11/RConn1 -- PhaseCswitch/RConn1
  PhaseCswitch/LConn1 -- Simscape Bus/LConn1
  PhaseCswitch/LConn2 -- Simscape Bus/LConn2
  PhaseBswitch/LConn1 -- Simscape Bus/LConn3
  PhaseBswitch/LConn2 -- Simscape Bus/LConn4
  PhaseAswitch/LConn1 -- Simscape Bus/LConn5
  PhaseAswitch/LConn2 -- Simscape Bus/LConn6

== system MotorDriveThermalTestbench/Motor Cooling/windingOilJet/ThermalResistance  ==
  "    HeatTransferCoefficient" : Subsystem
  Nusselt No : Subsystem
  Oil Wet Area : Subsystem
  PS Math Function : fl_lib/Physical Signals/Functions/PS Math Function  fcn_choice=foundation.enum.math_function.reciprocal  v=1
  PS Product : fl_lib/Physical Signals/Functions/PS Product
  PrNo : fl_lib/Physical Signals/Sources/PS Constant  constant=electricDrive.MotorThermal.Pr
  ReynoldsNo : Subsystem
  avgDriftVelocity : Subsystem
  FilmThickness : PMIOPort  Side=Left
  OD : PMIOPort  Port=2  Side=Left
  RTh : PMIOPort  Port=3  Side=Right
  Oil_flow : PMIOPort  Port=4  Side=Right
  connections:
  avgDriftVelocity/RConn1 -- ReynoldsNo/LConn1 -- Oil Wet Area/LConn3
  ReynoldsNo/LConn2 -- OD/RConn1 -- avgDriftVelocity/LConn1 -- "    HeatTransferCoefficient"/LConn2 -- Oil Wet Area/LConn4
  PrNo/RConn1 -- Nusselt No/LConn2
  "    HeatTransferCoefficient"/RConn1 -- PS Product/LConn2
  ReynoldsNo/RConn1 -- Nusselt No/LConn1
  Nusselt No/RConn1 -- "    HeatTransferCoefficient"/LConn1
  PS Math Function/RConn1 -- RTh/RConn1
  Oil Wet Area/RConn1 -- PS Product/LConn1
  PS Math Function/LConn1 -- PS Product/RConn1
  Oil_flow/RConn1 -- Oil Wet Area/LConn1
  FilmThickness/RConn1 -- Oil Wet Area/LConn2

== system MotorDriveThermalTestbench/Test Env N Controls/Motor speed N test environment/Motor Speed Reference ==
  VSpd : Inport  Unit=km/hr
  Constant1 : Constant  Value=electricDrive.VehicleParams.wheel_radius
  Constant2 : Constant  Value=electricDrive.VehicleParams.Gear_ratio
  Divide : Product  Inputs=*/
  Gain : Gain  Gain=2*pi
  Product : Product
  Signal Specification : SignalSpecification  Unit=m/min
  Unit Conversion : UnitConversion
  MtrSpdRef : Outport  Unit=rpm  VectorParamsAs1DForOutWhenUnconnected=off
  wires:
  VSpd/1 -> Unit Conversion/1
  Unit Conversion/1 -> Signal Specification/1
  Signal Specification/1 -> Divide/1
  Gain/1 -> Divide/2  "2*pi*R (m)"
  Divide/1 -> Product/1  "tireRpmRef"
  Constant2/1 -> Product/2
  Product/1 -> MtrSpdRef/1  "motorRpmRef"
  Constant1/1 -> Gain/1  "m"

== system MotorDriveThermalTestbench/Test Env N Controls/Motor speed N test environment/Test Environment ==
  tgtVspd : Inport
  Setting : Subsystem
  Transfer Fcn : TransferFcn  Numerator=[1 1]  Denominator=[0.1 1]
  BrakeSig : Outport
  wires:
  tgtVspd/1 -> Transfer Fcn/1
  Transfer Fcn/1 -> Setting/1(dec)
  Setting/1(b) -> BrakeSig/1

== system MotorDriveThermalTestbench/EM/Temperature/Rotor Thermal Block/Sensor ==
  Temperature Sensor : fl_lib/Thermal/Thermal Sensors/Temperature Sensor  temperature_measure=foundation.enum.MeasurementReference.difference
  Thermal Reference1 : fl_lib/Thermal/Thermal Elements/Thermal Reference
  " " : PMIOPort  Side=Left
  "  " : PMIOPort  Port=2  Side=Right
  connections:
  Temperature Sensor/LConn1 -- " "/RConn1
  Thermal Reference1/LConn1 -- Temperature Sensor/RConn1
  "  "/RConn1 -- Temperature Sensor/RConn2

== system MotorDriveThermalTestbench/EM/Temperature/Stator Thermal Block/Loss Correction ==
  PS Add : fl_lib/Physical Signals/Functions/PS Add
  PS Product : fl_lib/Physical Signals/Functions/PS Product
  PS Subtract : fl_lib/Physical Signals/Functions/PS Subtract
  Ref Temp Of loss calculations : fl_lib/Physical Signals/Sources/PS Constant  constant=298 K
  add 1 : fl_lib/Physical Signals/Sources/PS Constant  constant=1
  joule coefficient : fl_lib/Physical Signals/Functions/PS Gain  gain=0.00386 1/K
  I2R_Loss : PMIOPort  Side=Left
  Temp : PMIOPort  Port=2  Side=Left
  HCorrect : PMIOPort  Port=3  Side=Right
  connections:
  HCorrect/RConn1 -- PS Product/RConn1
  PS Subtract/RConn1 -- joule coefficient/LConn1
  joule coefficient/RConn1 -- PS Add/LConn1
  PS Add/RConn1 -- PS Product/LConn1
  I2R_Loss/RConn1 -- PS Product/LConn2
  Temp/RConn1 -- PS Subtract/LConn1
  Ref Temp Of loss calculations/RConn1 -- PS Subtract/LConn2
  add 1/RConn1 -- PS Add/LConn2

== system MotorDriveThermalTestbench/EM/Temperature/Stator Thermal Block/Sensor ==
  Temperature Sensor : fl_lib/Thermal/Thermal Sensors/Temperature Sensor  temperature_measure=foundation.enum.MeasurementReference.difference
  Thermal Reference1 : fl_lib/Thermal/Thermal Elements/Thermal Reference
  "  " : PMIOPort  Side=Left
  " " : PMIOPort  Port=2  Side=Right
  connections:
  " "/RConn1 -- Temperature Sensor/LConn1
  Temperature Sensor/RConn2 -- "  "/RConn1
  Thermal Reference1/LConn1 -- Temperature Sensor/RConn1

== system MotorDriveThermalTestbench/Inverter/AbstractInverter /Inverter Power Module Thermal/BasePLT ==
  Casing mass : fl_lib/Thermal/Thermal Elements/Thermal Mass  mass_type=foundation.enum.constant_variable.constant  mass=CaseParams.Mass kg  sp_heat=CaseParams.SpHeat J/(K*kg)  mass_min=1e-6 kg  num_ports=foundation.enum.numPorts2.one  m_specify=off  m_priority=High  m=1 kg  m_nominal_specify=off  m_nominal_value=1  m_nominal_unit=kg  T_specify=on  T_priority=High  T=electricDrive.PMparams.TinitCase K  T_nominal_specify=off  T_nominal_value=1  T_nominal_unit=K  Q_specify=off  Q_priority=None  Q=0 W  Q_nominal_specify=off  Q_nominal_value=1  Q_nominal_unit=W
  Conductive Heat Transfer : fl_lib/Thermal/Thermal Elements/Conductive Heat Transfer  thermal_type=foundation.enum.ConstantVariableTabulated.Constant  wall_geometry=foundation.enum.ConductionWallGeometry.Planar  area=CaseParams.Area m^2  thickness=CaseParams.Thickness m  d_in=0.05 m  d_out=0.1 m  L=1 m  th_cond_min=10 W/(K*m)  th_cond=CaseParams.SpHeat W/(K*m)  th_cond_TLU=[413, 401, 392, 383, 371, 357, 342] W/(K*m)  temp_TLU=[200, 273, 400, 600, 800, 1000, 1200] K  T_specify=off  T_priority=None  T=0 K  T_nominal_specify=off  T_nominal_value=1  T_nominal_unit=K  Q_specify=off  Q_priority=None  Q=0 W  Q_nominal_specify=off  Q_nominal_value=1  Q_nominal_unit=W
  Hinv : PMIOPort  Side=Left
  H : PMIOPort  Port=2  Side=Right
  connections:
  Conductive Heat Transfer/LConn1 -- Hinv/RConn1
  Casing mass/LConn1 -- H/RConn1 -- Conductive Heat Transfer/RConn1
